simulink model "blockdemo"  (Simulink 6.3)
settings: Solver=VariableStepDiscrete  StartTime=0  StopTime=8  RelTol=1e-3
InitFcn:
  | %% DSPBuilder Start
  | alt_dspbuilder_update_model(bdroot)
  | %% DSPBuilder End
libraries: allblocks_alteradspbuilder2 x15
settings Model: Creator=mjervis  LastModifiedBy=delphick
settings DataIOCC: SignalLoggingName=sigsOut
settings OptimizationCC: BlockReduction=off  BooleanDataType=off  InlineInvariantSignals=on
settings DebuggingCC: SolverPrmCheckMsg=none
settings HardwareCC: TargetUnknown=on

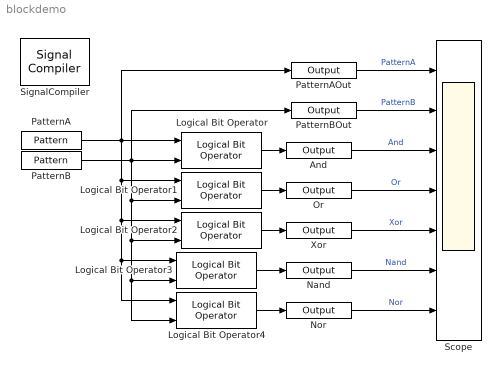
== system blockdemo ==
  And : allblocks_alteradspbuilder2/Output  iofile=C:\workspace_clean\Documentation\DesignExamples\Tutorials\UnitBlocks\GateAndControl\LogicalBitOperator\tb_blockdemo\blockdemo_And.capture  BusType=Single Bit  bwl=8  bwr=0  PORTTYPE=Output
  Logical Bit Operator : allblocks_alteradspbuilder2/Logical Bit Operator  LogicalOperator=AND  user_inputs=2
  Logical Bit Operator1 : allblocks_alteradspbuilder2/Logical Bit Operator  LogicalOperator=OR  user_inputs=2
  Logical Bit Operator2 : allblocks_alteradspbuilder2/Logical Bit Operator  LogicalOperator=XOR  user_inputs=2
  Logical Bit Operator3 : allblocks_alteradspbuilder2/Logical Bit Operator  LogicalOperator=NAND  user_inputs=2
  Logical Bit Operator4 : allblocks_alteradspbuilder2/Logical Bit Operator  LogicalOperator=NOR  user_inputs=2
  Nand : allblocks_alteradspbuilder2/Output  iofile=C:\workspace_clean\Documentation\DesignExamples\Tutorials\UnitBlocks\GateAndControl\LogicalBitOperator\tb_blockdemo\blockdemo_Nand.capture  BusType=Single Bit  bwl=8  bwr=0  PORTTYPE=Output
  Nor : allblocks_alteradspbuilder2/Output  iofile=C:\workspace_clean\Documentation\DesignExamples\Tutorials\UnitBlocks\GateAndControl\LogicalBitOperator\tb_blockdemo\blockdemo_Nor.capture  BusType=Single Bit  bwl=8  bwr=0  PORTTYPE=Output
  Or : allblocks_alteradspbuilder2/Output  iofile=C:\workspace_clean\Documentation\DesignExamples\Tutorials\UnitBlocks\GateAndControl\LogicalBitOperator\tb_blockdemo\blockdemo_Or.capture  BusType=Single Bit  bwl=8  bwr=0  PORTTYPE=Output
  PatternA : allblocks_alteradspbuilder2/Pattern  Sequence=00111111  SpecifyClock=off  use_ena=off  use_sclr=off
  PatternAOut : allblocks_alteradspbuilder2/Output  iofile=C:\workspace_clean\Documentation\DesignExamples\Tutorials\UnitBlocks\GateAndControl\LogicalBitOperator\tb_blockdemo\blockdemo_PatternAOut.capture  BusType=Single Bit  bwl=8  bwr=0  PORTTYPE=Output
  PatternB : allblocks_alteradspbuilder2/Pattern  Sequence=11111100  SpecifyClock=off  use_ena=off  use_sclr=off
  PatternBOut : allblocks_alteradspbuilder2/Output  iofile=C:\workspace_clean\Documentation\DesignExamples\Tutorials\UnitBlocks\GateAndControl\LogicalBitOperator\tb_blockdemo\blockdemo_PatternBOut.capture  BusType=Single Bit  bwl=8  bwr=0  PORTTYPE=Output
  Scope : Scope  NumInputPorts=7
      settings: TimeRange=8  YMin=-0.5~-0.5~-0.5~-0.5~-0.5~-0.5~-0.5  YMax=1.5~1.5~1.5~1.5~1.5~1.5~1.5  SampleInput=on  SampleTime=1
  SignalCompiler : allblocks_alteradspbuilder2/Signal Compiler  DeviceFamily=Stratix IV  DeviceName=AUTO  EnableSignalTap=off  SignalTapDepth=128  UseBoardBlock=off  StpUseDefaultClock=on  StpClock=clock
  Xor : allblocks_alteradspbuilder2/Output  iofile=C:\workspace_clean\Documentation\DesignExamples\Tutorials\UnitBlocks\GateAndControl\LogicalBitOperator\tb_blockdemo\blockdemo_Xor.capture  BusType=Single Bit  bwl=8  bwr=0  PORTTYPE=Output
  wires:
  Logical Bit Operator/1 -> And/1
  PatternA/1 -> PatternAOut/1, Logical Bit Operator/1, Logical Bit Operator1/1, Logical Bit Operator2/1, Logical Bit Operator3/1, Logical Bit Operator4/1
  PatternAOut/1 -> Scope/1  "PatternA"
  PatternB/1 -> PatternBOut/1, Logical Bit Operator/2, Logical Bit Operator1/2, Logical Bit Operator2/2, Logical Bit Operator3/2, Logical Bit Operator4/2
  PatternBOut/1 -> Scope/2  "PatternB"
  And/1 -> Scope/3  "And"
  Logical Bit Operator1/1 -> Or/1
  Logical Bit Operator2/1 -> Xor/1
  Logical Bit Operator3/1 -> Nand/1
  Logical Bit Operator4/1 -> Nor/1
  Nor/1 -> Scope/7  "Nor"
  Nand/1 -> Scope/6  "Nand"
  Xor/1 -> Scope/5  "Xor"
  Or/1 -> Scope/4  "Or"
